simulink model "CAR_SIM"  (R2022a)
settings: Solver=ode23t  StartTime=0.0  StopTime=100  MaxStep=1e-2  RelTol=1e-3
values from neighbouring files (symbols this model uses):
  Aobs = A    [Observer_Motor_PI.m]
  Buobs = Bu    [Observer_Motor_PI.m]
  Cobs = C    [Observer_Motor_PI.m]
  Klat =     [controllers.mat]
  Klong =     [controllers.mat]
  Lobs = inv(Gv)'*Yv    [Observer_Motor_PI.m]    (also in controllers.mat = [0.879044480997 -0.0788103412345 -0.879049416379 0.082382757)
  Psi0 = -pi/2    (= -1.57079632679)    [INIT_Calpha.m]    (also in INIT_Calpha_MPC.m)
  Servo = series(delay,c2d(Servo,Ts))    [BuildGridCustomSFGridDelay.m]    (also in INIT_Calpha.m; INIT_Calpha_MPC.m)
  tp = 0.95    [INIT_Calpha.m]    (also in INIT_Calpha_MPC.m)
  Ts = 1/50    (= 0.02)    [BuildGridCustomLongSF.m]    (also in BuildGridCustomSFGridDelay.m; DOFcontrMotor.m; INIT_Calpha.m; INIT_Calpha_MPC.m)
  v0 = 1    [INIT_Calpha.m]    (also in INIT_Calpha_MPC.m)
  vref = 1.5    [INIT_Calpha.m]    (also in INIT_Calpha_MPC.m = 1)
  Welat = We    [BuildGridCustomSFGridDelay.m]
  Welong = We    [BuildGridCustomLongSF.m]
  Wulat = Wu    [BuildGridCustomSFGridDelay.m]
  Wulong = Wu    [BuildGridCustomLongSF.m]
  x = [1 1 1 1]'    [Chat_K.m]    (also in xmotor.mat = [2.447723549e-05 2.93934049507 0.00376946337601 3.4220417427)
  X0 = Track.X(1)    [INIT_Calpha.m]    (also in INIT_Calpha_MPC.m)
  Y0 = Track.Y(1)    [INIT_Calpha.m]    (also in INIT_Calpha_MPC.m)
undefined symbols (not defined in the file or in its folder): GridKLong, Obs, Problem, purePursuitRefGen, Sched_K, simNLPVCalpha, Track
libraries: simulink x8, cstblocks x5
settings Model: Creator=ariel  LastModifiedBy=arielmedero
settings DebuggingCC: UnconnectedInputMsg=warning  UnconnectedOutputMsg=warning  UnconnectedLineMsg=warning
settings RTWCC: DLArmComputeVersion=19.05

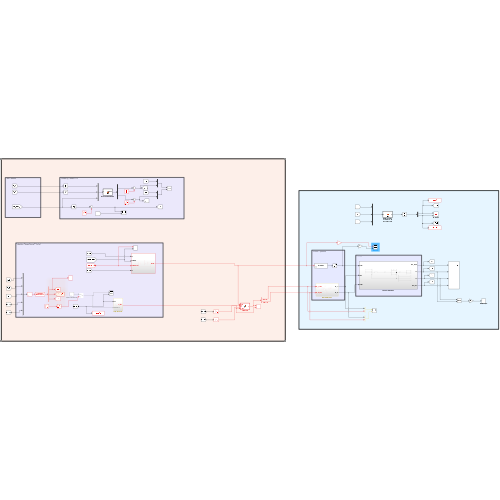
[thumbnail: Simulink's stored preview of the top-level diagram]
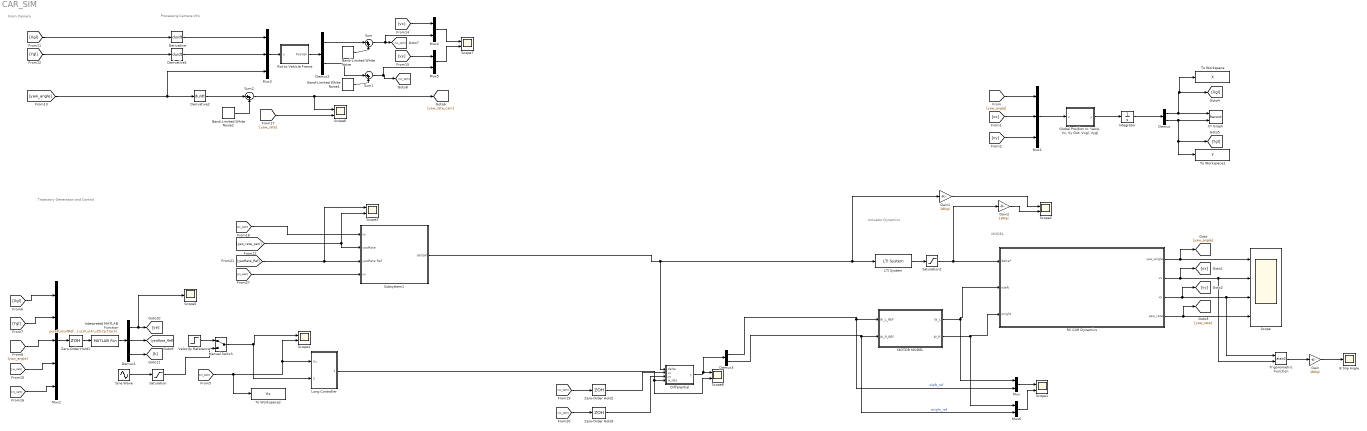
== system CAR_SIM ==
  note: MODEL
  note: Actuator Dynamics
  note: Trajectory Generation and Control
  note: Processing Camera Info
  note: From Camera
  B Slip Angle : Scope
  Band-Limited White Noise : simulink/Sources/Band-Limited White Noise  Cov=[0.000005]  Ts=Ts  seed=[23341]
  Band-Limited White Noise1 : simulink/Sources/Band-Limited White Noise  Cov=[0.0000025]  Ts=Ts  seed=[23341]
  Band-Limited White Noise2 : simulink/Sources/Band-Limited White Noise  Cov=[0.0001]  Ts=Ts  seed=[23341]
  Demux : Demux  Outputs=2
  Demux1 : Demux  Outputs=3
  Demux2 : Demux  Outputs=2
  Demux3 : Demux  Outputs=2
  Derivative : Derivative
  Derivative1 : Derivative
  Derivative2 : Derivative
  Differential : MATLAB Function  TreatAsAtomicUnit=on
  Gain : Gain  Gain=180/pi
  Gain1 : Gain  Gain=180/pi
  Gain2 : Gain  Gain=180/pi
  "Global Position In: YawA, Vx, Vy Out: Vxgl, Vygl" : MATLAB Function  TreatAsAtomicUnit=on
  Integrator : Integrator  InitialCondition=[X0,Y0]
  Interpreted MATLAB Function : MATLABFcn  MATLABFcn=purePursuitRefGen(u(1),u(2),u(3),u(4),u(5),tp,Track)  OutputDimensions=3
  LTI System : cstblocks/LTI System  sys=servoSIM  IC=[]
  Long Controller : Subsystem
  MOTOR MODEL : Subsystem
  Manual Switch : ManualSwitch
  Mux{,4..6} (4 alike) : Mux  Inputs=2
  Mux1 : Mux  Inputs=3
  Mux2 : Mux  Inputs=5
  Mux3 : Mux  Inputs=3
  RC CAR Dynamics : Subsystem
  Rot to Vehicle Frame : MATLAB Function  TreatAsAtomicUnit=on
  Saturation : Saturate  UpperLimit=2  LowerLimit=0.5
  Saturation2 : Saturate  UpperLimit=0.7  LowerLimit=-0.7
  Scope : Scope  NumInputPorts=4
  Scope{1..4,6..8} (7 alike) : Scope  NumInputPorts=2
  Scope5 : Scope
  Sine Wave : Sin  Amplitude=0.3  Bias=vref  Frequency=2*pi*(1/10)  SampleTime=Ts
  Subsystem1 : Subsystem
  Sum : Sum  Inputs=|++
  Sum1 : Sum  Inputs=|++
  Sum2 : Sum  Inputs=|++
  To Workspace : ToWorkspace  VariableName=X  SampleTime=Ts
      settings: Decimation=3
  To Workspace1 : ToWorkspace  VariableName=Y  SampleTime=Ts
      settings: Decimation=3
  To Workspace2 : ToWorkspace  VariableName=Vx  SampleTime=Ts
      settings: Decimation=3
  Trigonometric Function : Trigonometry  Operator=atan2
  Velocity Reference : Step  Time=30  Before=vref  After=vref  SampleTime=0
  XY Graph : Record  FileSettingsInternal="{\"entries\":[{\"content\":{\"excelSettings\":{\"content\":{},\"type\":\"Streamout.ExcelSettings\"}},\"type\":\"Streamout.FileSettingStorage\",\"uuid\":\"be3c7d72-63e6-4d9c-a37d-d5c7a5cbb730\"}],\"packageUris\":[\"http://schema.mathworks.com/mf0/streamout_blocks/R2020a\"],\"version\":\"1.0\"}"  Layout=[1 1]  SignalsInternal="{\"entries\":[{\"content\":{\"signals\":[{\"content\":{\"blockPath\":[\"CAR_SIM/XY Graph\"],\"channel\":[],\"dimensions\":[1],\"domain\":\"CAR_SIM/XY Graph\",\"lineColor\":\"#b746ff\",\"plots\":[],\"port\":1,\"sid\":[\"\"],\"signalID\":96,\"signalName\":\"Demux:1\"},\"type\":\"RecordBlkView.Signal\",\"uuid\":\"d8c3de26-eb54-467e-8f7c-a31bb6b0b039\"},{\"content\":{\"blockPath\":[\"CAR_SIM/XY Graph\"],\"channel\":[],\"dimensions\":[1],\"domain\":\"CAR_SIM/XY Graph\",\"lineColor\":\"#64d413\",\"plots\":[],\"port\":2,\"sid\":[\"\"],\"signalID\":100,\"signalName\":\"Demux:2\"},\"type\":\"RecordBlkView.Signal\",\"uuid\":\"63afb63a-788f-4590-beec-63754803458f\"}]},\"type\":\"RecordBlkView.InputSignals\",\"uuid\":\"599c7bf7-74eb-4bb7-9e4f-c575138a6709\"}],\"packageUris\":[\"http://schema.mathworks.com/mf0/streamout_blocks/R2020a\"],\"version\":\"1.0\"}"  VisualizationBindings="{\"xyplotplugin\":{\"info\":[{\"series\":[],\"subplotID\":1}]}}"  CompatibilityTag=XY
  Zero-Order Hold1 : ZeroOrderHold  SampleTime=Ts
  Zero-Order Hold2 : ZeroOrderHold  SampleTime=Ts
  Zero-Order Hold3 : ZeroOrderHold  SampleTime=Ts
  wires:
  Mux1/1 -> "Global Position In: YawA, Vx, Vy Out: Vxgl, Vygl"/1(u)
  RC CAR Dynamics/1(yaw_angle) -> Scope/1, [yaw_angle]
  RC CAR Dynamics/2(vx) -> Trigonometric Function/2, Scope/2, [vx]
  RC CAR Dynamics/3(vy) -> Trigonometric Function/1, Scope/3, [vy]
  RC CAR Dynamics/4(yaw_rate) -> Scope/4, [yaw_rate]
  [yaw_angle] -> Mux1/1
  [vx] -> Mux1/2
  [vy] -> Mux1/3
  "Global Position In: YawA, Vx, Vy Out: Vxgl, Vygl"/1(y) -> Integrator/1
  Integrator/1 -> Demux/1
  Demux/1 -> XY Graph/1, To Workspace/1, [Xgl]
  Demux/2 -> XY Graph/2, To Workspace1/1, [Ygl]
  Trigonometric Function/1 -> Gain/1
  Gain/1 -> B Slip Angle/1
  Long Controller/1(w_des) -> Scope8/2, Differential/4(w_des)
  [Xgl] -> Mux2/1
  [Ygl] -> Mux2/2
  [yaw_angle] -> Mux2/3
  [vx_cam] -> Mux2/4
  [vy_cam] -> Mux2/5
  [Xgl] -> Derivative/1
  [Ygl] -> Derivative1/1
  [yaw_angle] -> Mux3/3, Derivative2/1
  Mux3/1 -> Rot to Vehicle Frame/1(u)
  Rot to Vehicle Frame/1(PosVeh) -> Demux2/1
  Mux4/1 -> Scope7/1
  Mux5/1 -> Scope7/2
  [vx] -> Mux4/1
  Demux2/1 -> Sum/1
  [vy] -> Mux5/1
  [vx_cam] -> To Workspace2/1, Scope4/2, Long Controller/1(Vx)
  [yaw_rate] -> Scope6/2
  Mux2/1 -> Zero-Order Hold1/1
  Derivative/1 -> Mux3/1
  Derivative1/1 -> Mux3/2
  Zero-Order Hold1/1 -> Interpreted MATLAB Function/1
  Gain1/1 -> Scope2/1
  Gain2/1 -> Scope2/2
  Demux3/2 -> Mux6/2, MOTOR MODEL/2(W_R_REF)  "wright_ref"
  Zero-Order Hold2/1 -> Differential/2(vx)
  Zero-Order Hold3/1 -> Differential/3(vy)
  [vx_cam] -> Zero-Order Hold2/1
  Differential/1(y) -> Demux3/1, Scope8/1
  Demux3/1 -> Mux/2, MOTOR MODEL/1(W_L_REF)  "wleft_ref"
  [vy_cam] -> Zero-Order Hold3/1
  Mux/1 -> Scope1/1
  Mux6/1 -> Scope1/2
  Saturation2/1 -> RC CAR Dynamics/1(delta*), Gain2/1
  MOTOR MODEL/1(W_L) -> RC CAR Dynamics/2(wleft), Mux/1
  MOTOR MODEL/2(W_R) -> RC CAR Dynamics/3(wright), Mux6/1
  Sum/1 -> Mux4/2, [vx_cam]
  Band-Limited White Noise/1 -> Sum/2
  Sum1/1 -> Mux5/2, [vy_cam]
  Demux2/2 -> Sum1/1
  Band-Limited White Noise1/1 -> Sum1/2
  Band-Limited White Noise2/1 -> Sum2/2
  Derivative2/1 -> Sum2/1
  Sum2/1 -> Scope6/1, [yaw_rate_cam]
  Manual Switch/1 -> Long Controller/2(Reference), Scope4/1
  Velocity Reference/1 -> Manual Switch/1
  Sine Wave/1 -> Saturation/1
  Saturation/1 -> Manual Switch/2
  Interpreted MATLAB Function/1 -> Demux1/1
  Demux1/2 -> [yawRate_Ref]
  Demux1/1 -> Scope5/1, [ye]
  Demux1/3 -> [k]
  LTI System/1 -> Saturation2/1
  [yaw_rate_cam] -> Scope3/2, Subsystem1/2(yawRate)
  [vx_cam] -> Subsystem1/4(vx)
  [vy_cam] -> Subsystem1/1(vy)
  [yawRate_Ref] -> Scope3/1, Subsystem1/3(yawRate Ref)
  Subsystem1/1(deltaK) -> Differential/1(delta), Gain1/1, LTI System/1

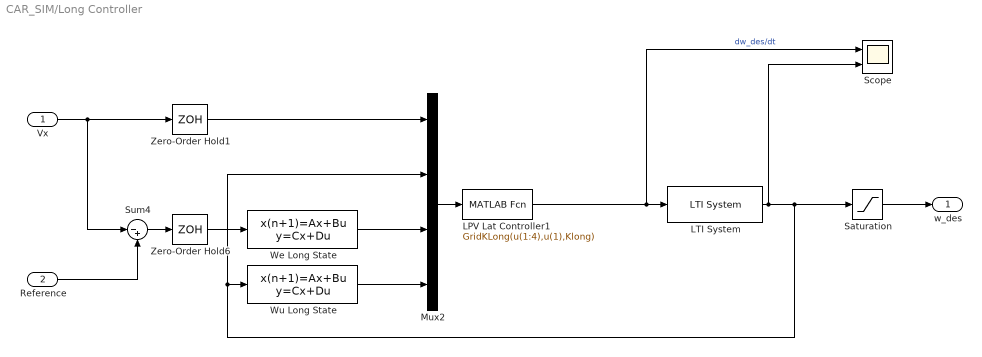
== system CAR_SIM/Long Controller ==
  Vx : Inport
  Reference : Inport  Port=2
  LPV Lat Controller1 : MATLABFcn  MATLABFcn=GridKLong(u(1:4),u(1),Klong)  OutputDimensions=1
  LTI System : cstblocks/LTI System  sys=Int  IC=[]
  Mux2 : Mux
  Saturation : Saturate  UpperLimit=100  LowerLimit=10
  Scope : Scope  NumInputPorts=2
  Sum4 : Sum  Inputs=|-+
  We Long State : DiscreteStateSpace  A=Welong.A  B=Welong.B  D=0  SampleTime=Ts
  Wu Long State : DiscreteStateSpace  A=Wulong.A  B=Wulong.B  D=0  SampleTime=Ts
  Zero-Order Hold1 : ZeroOrderHold  SampleTime=Ts
  Zero-Order Hold6 : ZeroOrderHold  SampleTime=Ts
  w_des : Outport
  wires:
  LPV Lat Controller1/1 -> Scope/1, LTI System/1  "dw_des/dt"
  Mux2/1 -> LPV Lat Controller1/1
  Zero-Order Hold1/1 -> Mux2/1
  Reference/1 -> Sum4/2
  Sum4/1 -> Zero-Order Hold6/1
  Vx/1 -> Sum4/1, Zero-Order Hold1/1
  Zero-Order Hold6/1 -> We Long State/1
  Saturation/1 -> w_des/1
  LTI System/1 -> Scope/2, Wu Long State/1, Mux2/2, Saturation/1
  Wu Long State/1 -> Mux2/4
  We Long State/1 -> Mux2/3

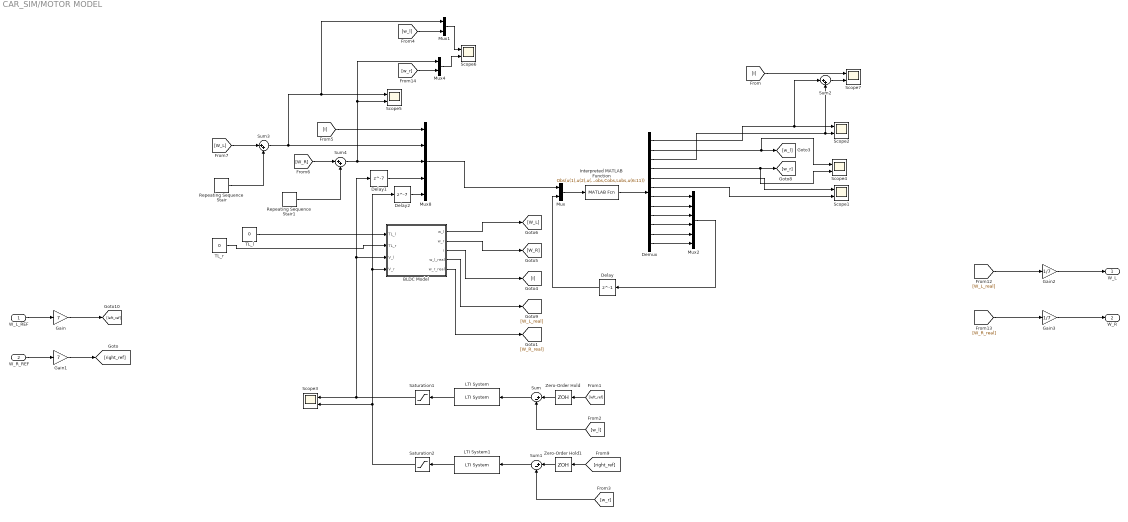
== system CAR_SIM/MOTOR MODEL ==
  W_L_REF : Inport
  W_R_REF : Inport  Port=2
  "BLDC Model " : Subsystem
  Delay : Delay  DelayLength=1  InitialCondition="[0 0 0 0  0 0]'"  SampleTime=Ts
  Delay1 : Delay  DelayLength=7  SampleTime=Ts
  Delay2 : Delay  DelayLength=7  SampleTime=Ts
  Demux : Demux  Outputs=12
  Gain : Gain  Gain=7
  Gain1 : Gain  Gain=7
  Gain2 : Gain  Gain=1/7
  Gain3 : Gain  Gain=1/7
  Interpreted MATLAB Function : MATLABFcn  MATLABFcn=Obs(u(1),u(2),u(3),u(4),u(5),Aobs,Buobs,Cobs,Lobs,u(6:11))  OutputDimensions=12
  LTI System : cstblocks/LTI System  sys=Kbldc  IC=[]
  LTI System1 : cstblocks/LTI System  sys=Kbldc  IC=[]
  Mux : Mux  Inputs=2
  Mux1 : Mux  Inputs=2
  Mux2 : Mux  Inputs=6
  Mux4 : Mux  Inputs=2
  Mux8 : Mux  Inputs=5
  Repeating Sequence Stair : simulink/Sources/Repeating Sequence Stair  OutValues=[0 0 0 0 0 0 0 0 0 0 0 0 0 0 0 0 0 0 0 0 0 0 0 0 0 0 0 0 0 0 0 0 0 0 0 0 0 0 0 0 800].'  tsamp=0.2  OutMin=[]  OutMax=[]  OutDataTypeStr=double  OutputDataTypeScalingMode=double  OutDataType=fixdt(0,8)  ConRadixGroup=Best Precision: Vector-wise  OutScaling=2^-12
  Repeating Sequence Stair1 : simulink/Sources/Repeating Sequence Stair  OutValues=[0 0 0 0 0 0 0 0 0 0 0 0 0 0 0 0 0 0 0 0 0 0 0 0 0 0 0 0 0 0 1000].'  tsamp=0.3  OutMin=[]  OutMax=[]  OutDataTypeStr=double  OutputDataTypeScalingMode=double  OutDataType=fixdt(0,8)  ConRadixGroup=Best Precision: Vector-wise  OutScaling=2^-12
  Saturation1 : Saturate  UpperLimit=1000  LowerLimit=0
  Saturation2 : Saturate  UpperLimit=1000  LowerLimit=0
  Scope{1..7} (7 alike) : Scope  NumInputPorts=2
  Sum : Sum  Inputs=|+-
  Sum1 : Sum  Inputs=|+-
  Sum2 : Sum  Inputs=|++
  Sum3 : Sum  Inputs=|++
  Sum4 : Sum  Inputs=|++
  TL_l : Constant  Value=0
  TL_r : Constant  Value=0
  Zero-Order Hold : ZeroOrderHold  SampleTime=Ts
  Zero-Order Hold1 : ZeroOrderHold  SampleTime=Ts
  W_L : Outport
  W_R : Outport  Port=2
  wires:
  "BLDC Model "/3(i) -> [I]
  TL_r/1 -> "BLDC Model "/2(TL_r)
  Mux2/1 -> Delay/1
  [I] -> Mux8/1
  "BLDC Model "/2(w_r) -> [W_R]
  "BLDC Model "/1(w_l) -> [W_L]
  TL_l/1 -> "BLDC Model "/1(TL_l)
  Demux/4 -> Scope4/2, [w_r]
  Delay/1 -> Mux/2
  Interpreted MATLAB Function/1 -> Demux/1
  Mux/1 -> Interpreted MATLAB Function/1
  Mux8/1 -> Mux/1
  "BLDC Model "/4(w_l_real) -> [W_L_real]
  "BLDC Model "/5(w_r_real) -> [W_R_real]
  [W_L_real] -> Gain2/1
  [W_R_real] -> Gain3/1
  W_L_REF/1 -> Gain/1
  W_R_REF/1 -> Gain1/1
  Gain/1 -> [left_ref]
  Gain1/1 -> [right_ref]
  Gain2/1 -> W_L/1
  Gain3/1 -> W_R/1
  Demux/7 -> Mux2/1
  Demux/8 -> Mux2/2
  Demux/9 -> Mux2/3
  Demux/10 -> Mux2/4
  Demux/11 -> Mux2/5
  Demux/12 -> Mux2/6
  Demux/5 -> Scope1/1
  Demux/6 -> Scope1/2
  Demux/1 -> Sum2/1, Scope2/1
  [W_L] -> Sum3/1
  Sum3/1 -> Mux1/1, Scope5/1, Mux8/2
  Repeating Sequence Stair/1 -> Sum3/2
  Demux/2 -> Scope4/1, [w_l]
  Repeating Sequence Stair1/1 -> Sum4/2
  [W_R] -> Sum4/1
  Sum4/1 -> Mux4/1, Scope5/2, Mux8/3
  Mux1/1 -> Scope6/1
  [w_l] -> Mux1/2
  Mux4/1 -> Scope6/2
  [w_r] -> Mux4/2
  LTI System/1 -> Saturation1/1
  LTI System1/1 -> Saturation2/1
  [left_ref] -> Zero-Order Hold/1
  Zero-Order Hold/1 -> Sum/1
  [w_l] -> Sum/2
  Sum/1 -> LTI System/1
  Sum1/1 -> LTI System1/1
  [right_ref] -> Zero-Order Hold1/1
  [w_r] -> Sum1/2
  Zero-Order Hold1/1 -> Sum1/1
  Delay1/1 -> Mux8/4
  Delay2/1 -> Mux8/5
  Demux/3 -> Sum2/2, Scope2/2
  Sum2/1 -> Scope7/2
  [I] -> Scope7/1
  Saturation1/1 -> Scope3/1, Delay1/1, "BLDC Model "/3(V_l)
  Saturation2/1 -> Scope3/2, Delay2/1, "BLDC Model "/4(V_r)

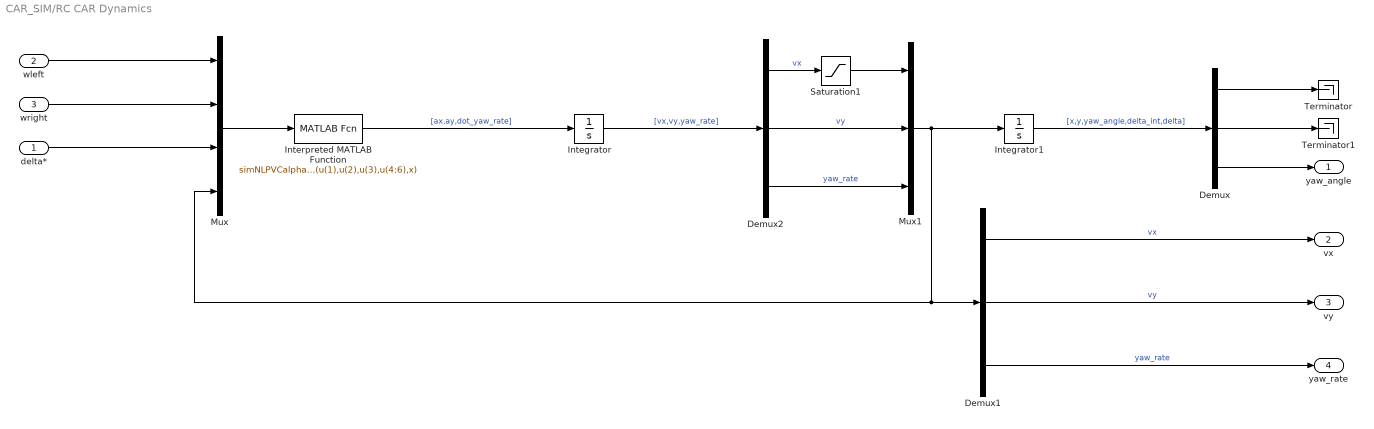
== system CAR_SIM/RC CAR Dynamics ==
  delta* : Inport
  wleft : Inport  Port=2
  wright : Inport  Port=3
  Demux : Demux  Outputs=3
  Demux1 : Demux  Outputs=3
  Demux2 : Demux  Outputs=3
  Integrator : Integrator  InitialCondition=[v0,0,0]
  Integrator1 : Integrator  InitialCondition=[0,0,Psi0]
  Interpreted MATLAB Function : MATLABFcn  MATLABFcn=simNLPVCalpha(u(1),u(2),u(3),u(4:6),x)  OutputDimensions=3
  Mux : Mux
  Mux1 : Mux  Inputs=3
  Saturation1 : Saturate  UpperLimit=1000  LowerLimit=0.1
  Terminator : Terminator
  Terminator1 : Terminator
  yaw_angle : Outport
  vx : Outport  Port=2
  vy : Outport  Port=3
  yaw_rate : Outport  Port=4
  wires:
  Integrator1/1 -> Demux/1  "[x,y,yaw_angle,delta_int,delta]"
  Demux/1 -> Terminator/1
  Demux/2 -> Terminator1/1
  Mux/1 -> Interpreted MATLAB Function/1
  Demux/3 -> yaw_angle/1
  Demux1/1 -> vx/1  "vx"
  Demux1/3 -> yaw_rate/1  "yaw_rate"
  Demux1/2 -> vy/1  "vy"
  wright/1 -> Mux/2
  wleft/1 -> Mux/1
  delta*/1 -> Mux/3
  Interpreted MATLAB Function/1 -> Integrator/1  "[ax,ay,dot_yaw_rate]"
  Demux2/3 -> Mux1/3  "yaw_rate"
  Mux1/1 -> Mux/4, Demux1/1, Integrator1/1
  Demux2/1 -> Saturation1/1  "vx"
  Demux2/2 -> Mux1/2  "vy"
  Integrator/1 -> Demux2/1  "[vx,vy,yaw_rate]"
  Saturation1/1 -> Mux1/1

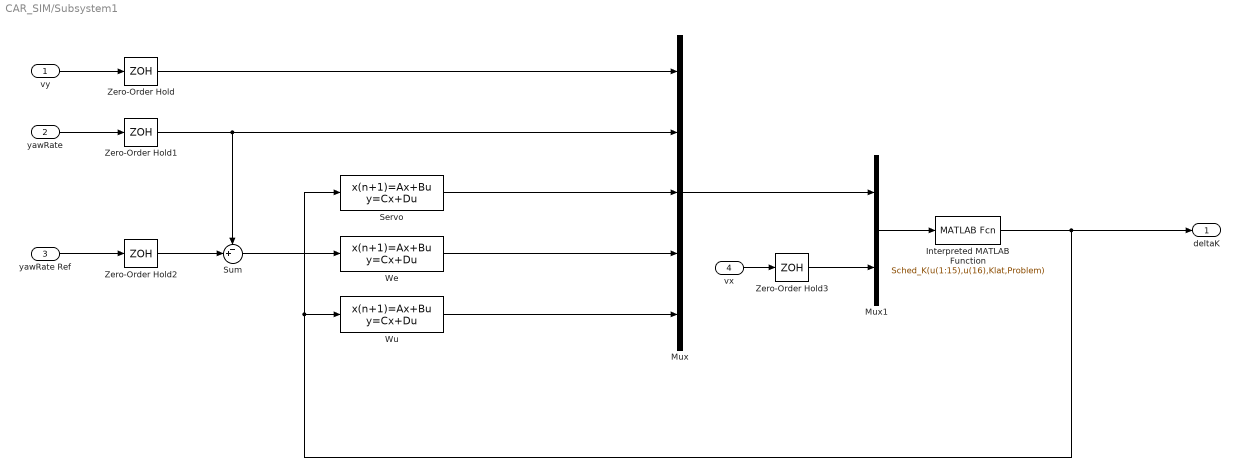
== system CAR_SIM/Subsystem1 ==
  vy : Inport
  yawRate : Inport  Port=2
  yawRate Ref : Inport  Port=3
  vx : Inport  Port=4
  Interpreted MATLAB Function : MATLABFcn  MATLABFcn=Sched_K(u(1:15),u(16),Klat,Problem)  OutputDimensions=1
  Mux : Mux  Inputs=5
  Mux1 : Mux  Inputs=2
  Servo : DiscreteStateSpace  A=Servo.A  B=Servo.B  C=eye(length(Servo.A))  D=zeros(length(Servo.A),1)  SampleTime=Ts
  Sum : Sum  Inputs=-+|
  We : DiscreteStateSpace  A=Welat.A  B=Welat.B  D=0  SampleTime=Ts
  Wu : DiscreteStateSpace  A=Wulat.A  B=Wulat.B  D=0  SampleTime=Ts
  Zero-Order Hold{,1..3} (4 alike) : ZeroOrderHold  SampleTime=Ts
  deltaK : Outport
  wires:
  vy/1 -> Zero-Order Hold/1
  yawRate/1 -> Zero-Order Hold1/1
  yawRate Ref/1 -> Zero-Order Hold2/1
  Zero-Order Hold/1 -> Mux/1
  Zero-Order Hold1/1 -> Mux/2, Sum/1
  Mux1/1 -> Interpreted MATLAB Function/1
  Mux/1 -> Mux1/1
  vx/1 -> Zero-Order Hold3/1
  Zero-Order Hold3/1 -> Mux1/2
  Zero-Order Hold2/1 -> Sum/2
  Wu/1 -> Mux/5
  Servo/1 -> Mux/3
  We/1 -> Mux/4
  Sum/1 -> We/1
  Interpreted MATLAB Function/1 -> Wu/1, Servo/1, deltaK/1

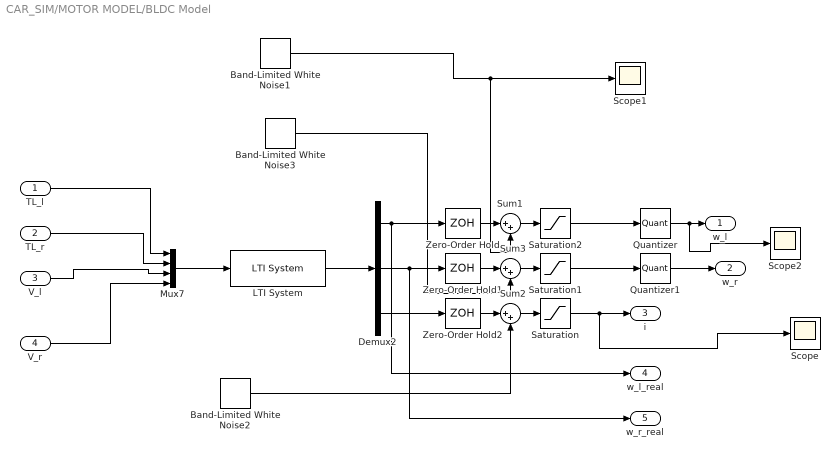
== system CAR_SIM/MOTOR MODEL/BLDC Model  ==
  TL_l : Inport
  TL_r : Inport  Port=2
  V_l : Inport  Port=3
  V_r : Inport  Port=4
  Band-Limited White Noise1 : simulink/Sources/Band-Limited White Noise  Cov=[150]  Ts=Ts  seed=[2381]
  Band-Limited White Noise2 : simulink/Sources/Band-Limited White Noise  Cov=[0.001]  Ts=Ts  seed=[235581]
  Band-Limited White Noise3 : simulink/Sources/Band-Limited White Noise  Cov=[170]  Ts=Ts  seed=[23666581]
  Demux2 : Demux  Outputs=3
  LTI System : cstblocks/LTI System  sys=Gmotor  IC=[0 0 0 0]
  Mux7 : Mux
  Quantizer : Quantizer  QuantizationInterval=70
  Quantizer1 : Quantizer  QuantizationInterval=70
  Saturation : Saturate  UpperLimit=1000  LowerLimit=0
  Saturation1 : Saturate  UpperLimit=1000  LowerLimit=0
  Saturation2 : Saturate  UpperLimit=1000  LowerLimit=0
  Scope : Scope
  Scope1 : Scope
  Scope2 : Scope
  Sum1 : Sum  Inputs=|++
  Sum2 : Sum  Inputs=|++
  Sum3 : Sum  Inputs=|++
  Zero-Order Hold : ZeroOrderHold  SampleTime=Ts
  Zero-Order Hold1 : ZeroOrderHold  SampleTime=Ts
  Zero-Order Hold2 : ZeroOrderHold  SampleTime=Ts
  w_l : Outport
  w_r : Outport  Port=2
  i : Outport  Port=3
  w_l_real : Outport  Port=4
  w_r_real : Outport  Port=5
  wires:
  LTI System/1 -> Demux2/1
  V_l/1 -> Mux7/3
  TL_r/1 -> Mux7/2
  V_r/1 -> Mux7/4
  Mux7/1 -> LTI System/1
  TL_l/1 -> Mux7/1
  Demux2/3 -> Zero-Order Hold2/1
  Band-Limited White Noise2/1 -> Sum2/2
  Sum2/1 -> Saturation/1
  Demux2/2 -> Zero-Order Hold1/1, w_r_real/1
  Demux2/1 -> Zero-Order Hold/1, w_l_real/1
  Quantizer/1 -> Scope2/1, w_l/1
  Quantizer1/1 -> w_r/1
  Saturation/1 -> Scope/1, i/1
  Zero-Order Hold2/1 -> Sum2/1
  Band-Limited White Noise1/1 -> Sum1/2, Scope1/1
  Zero-Order Hold/1 -> Sum1/1
  Sum1/1 -> Saturation2/1
  Sum3/1 -> Saturation1/1
  Zero-Order Hold1/1 -> Sum3/1
  Band-Limited White Noise3/1 -> Sum3/2
  Saturation1/1 -> Quantizer1/1
  Saturation2/1 -> Quantizer/1

== matlab function CAR_SIM/Global Position In: YawA, Vx, Vy Out: Vxgl, Vygl ==
  data: u input; y output
function y = fcn(u)
    phi = u(1);
    Vx = u(2);
    Vy = u(3);
    beta = atan(Vy/Vx);
    V = sqrt(Vx^2+Vy^2);
    
    Xd = V*cos(phi+beta);
    Yd = V*sin(phi+beta);
    
y = [Xd;Yd];

== matlab function CAR_SIM/Rot to Vehicle Frame ==
  data: u input; PosVeh output
function PosVeh = fcn(u)

Xgl = u(1);
Ygl = u(2);
psi = u(3);

Pos = [Xgl Ygl]';
R = [cos(psi) -sin(psi);sin(psi) cos(psi)]';
PosVeh = R*Pos;


end

== matlab function CAR_SIM/Differential ==
  data: delta input; vx input; vy input; y output; w_des input
function y = fcn(delta,vx,vy,w_des)
%Car Parameters

    L=0.174; % length of the car
    Wi=0.087; % width of the car
    R = 0.031631112759405; %  Wheel radius


    v = norm([vx vy]); 
    delta_w = (Wi/2)*v*tan(delta)/(L*R);
    w_l = w_des-delta_w/2;
    w_r = w_des+delta_w/2;
    y = [w_l,w_r];
